simulink model "Code_Gen_Model"  (R2023b)
settings: Solver=FixedStepDiscrete  StartTime=0.0  StopTime=inf  FixedStep=t_sample  RelTol=1e-3
settings Model: Creator=FIRSTMentor
settings OptimizationCC: DefaultParameterBehavior=Inlined  StrengthReduction=on  PassReuseOutputArgsAs=Individual arguments  ZeroExternalMemoryAtStartup=off  ZeroInternalMemoryAtStartup=off  OptimizeBlockOrder=speed  OptimizationPriority=Speed  OptimizationCustomize=off  MultiThreadedLoops=on  EfficientTunableParamExpr=on
settings DebuggingCC: MergeDetectMultiDrivingBlocksExec=none  ParameterTunabilityLossMsg=error
settings ModelReferenceCC: PropagateSignalLabelsOutOfModel=off
settings SFSimCC: MATLABDynamicMemAlloc=off
settings RTWCC: Description=Embedded Coder  SystemTargetFile=ert.tlc  GenCodeOnly=on  TemplateMakefile=ert_default_tmf  Toolchain=MinGW64 | gmake (64-bit Windows)
settings CodeAppCC: ForceParamTrailComments=on  IgnoreCustomStorageClasses=off  OperatorAnnotations=on  SimulinkDataObjDesc=on  SFDataObjDesc=on  InsertBlockDesc=on
settings ERTTargetCC: TargetLangStandard=C99 (ISO)  GenerateSampleERTMain=on  ParenthesesLevel=Minimum  InlinedParameterPlacement=NonHierarchical  ERTCustomFileTemplate=example_file_process.tlc

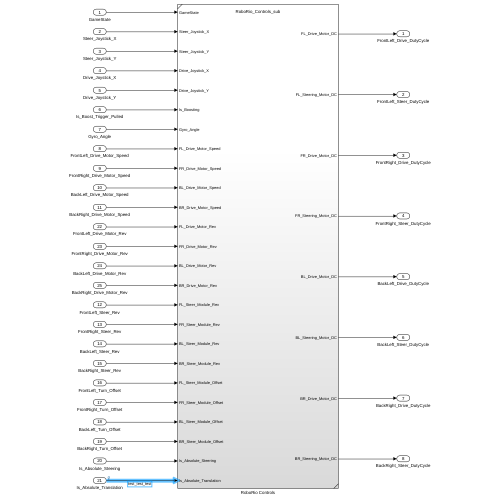
[thumbnail: Simulink's stored preview of the top-level diagram]
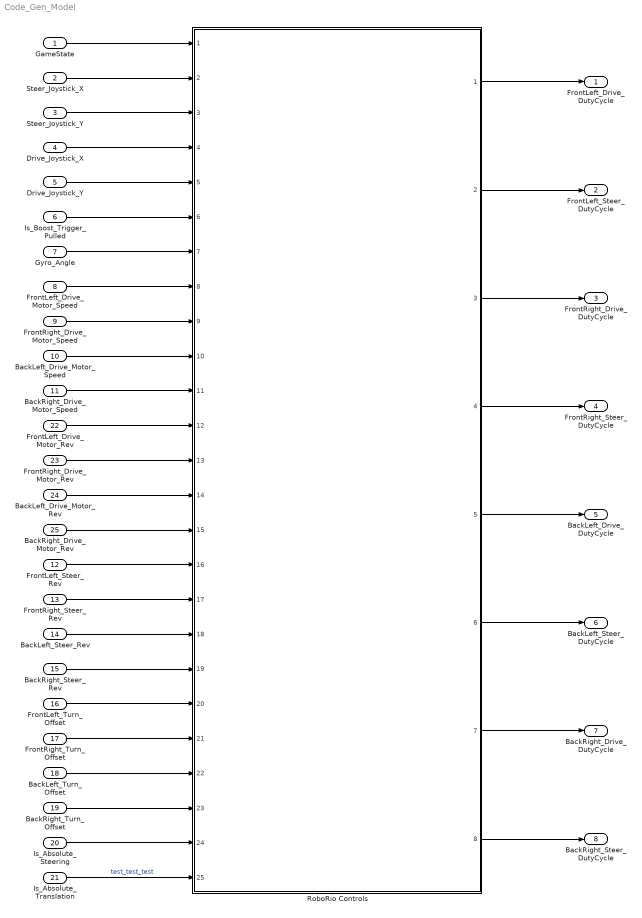
== system Code_Gen_Model ==
  GameState : Inport
  Steer_Joystick_X : Inport  Port=2
  Steer_Joystick_Y : Inport  Port=3
  Drive_Joystick_X : Inport  Port=4
  Drive_Joystick_Y : Inport  Port=5
  Is_Boost_Trigger_Pulled : Inport  Port=6
  Gyro_Angle : Inport  Port=7
  FrontLeft_Drive_Motor_Speed : Inport  Port=8
  FrontRight_Drive_Motor_Speed : Inport  Port=9
  BackLeft_Drive_Motor_Speed : Inport  Port=10
  BackRight_Drive_Motor_Speed : Inport  Port=11
  FrontLeft_Steer_Rev : Inport  Port=12
  FrontRight_Steer_Rev : Inport  Port=13
  BackLeft_Steer_Rev : Inport  Port=14
  BackRight_Steer_Rev : Inport  Port=15
  FrontLeft_Turn_Offset : Inport  Port=16
  FrontRight_Turn_Offset : Inport  Port=17
  BackLeft_Turn_Offset : Inport  Port=18
  BackRight_Turn_Offset : Inport  Port=19
  Is_Absolute_Steering : Inport  Port=20
  Is_Absolute_Translation : Inport  Port=21
  FrontLeft_Drive_Motor_Rev : Inport  Port=22
  FrontRight_Drive_Motor_Rev : Inport  Port=23
  BackLeft_Drive_Motor_Rev : Inport  Port=24
  BackRight_Drive_Motor_Rev : Inport  Port=25
  RoboRio Controls : Subsystem  ReferencedSubsystem=RoboRio_Controls_sub
  FrontLeft_Drive_DutyCycle : Outport
  FrontLeft_Steer_DutyCycle : Outport  Port=2
  FrontRight_Drive_DutyCycle : Outport  Port=3
  FrontRight_Steer_DutyCycle : Outport  Port=4
  BackLeft_Drive_DutyCycle : Outport  Port=5
  BackLeft_Steer_DutyCycle : Outport  Port=6
  BackRight_Drive_DutyCycle : Outport  Port=7
  BackRight_Steer_DutyCycle : Outport  Port=8
  wires:
  RoboRio Controls/7 -> BackRight_Drive_DutyCycle/1
  Drive_Joystick_X/1 -> RoboRio Controls/4
  Is_Absolute_Steering/1 -> RoboRio Controls/24
  Steer_Joystick_X/1 -> RoboRio Controls/2
  RoboRio Controls/3 -> FrontRight_Drive_DutyCycle/1
  BackRight_Turn_Offset/1 -> RoboRio Controls/23
  GameState/1 -> RoboRio Controls/1
  RoboRio Controls/4 -> FrontRight_Steer_DutyCycle/1
  Is_Boost_Trigger_Pulled/1 -> RoboRio Controls/6
  FrontLeft_Drive_Motor_Speed/1 -> RoboRio Controls/8
  RoboRio Controls/6 -> BackLeft_Steer_DutyCycle/1
  BackLeft_Steer_Rev/1 -> RoboRio Controls/18
  Gyro_Angle/1 -> RoboRio Controls/7
  FrontRight_Steer_Rev/1 -> RoboRio Controls/17
  Steer_Joystick_Y/1 -> RoboRio Controls/3
  Drive_Joystick_Y/1 -> RoboRio Controls/5
  RoboRio Controls/2 -> FrontLeft_Steer_DutyCycle/1
  FrontRight_Drive_Motor_Speed/1 -> RoboRio Controls/9
  BackLeft_Drive_Motor_Speed/1 -> RoboRio Controls/10
  BackLeft_Turn_Offset/1 -> RoboRio Controls/22
  BackRight_Drive_Motor_Speed/1 -> RoboRio Controls/11
  FrontLeft_Drive_Motor_Rev/1 -> RoboRio Controls/12
  Is_Absolute_Translation/1 -> RoboRio Controls/25  "test_test_test"
  BackRight_Steer_Rev/1 -> RoboRio Controls/19
  FrontRight_Drive_Motor_Rev/1 -> RoboRio Controls/13
  BackLeft_Drive_Motor_Rev/1 -> RoboRio Controls/14
  BackRight_Drive_Motor_Rev/1 -> RoboRio Controls/15
  FrontLeft_Steer_Rev/1 -> RoboRio Controls/16
  RoboRio Controls/8 -> BackRight_Steer_DutyCycle/1
  FrontLeft_Turn_Offset/1 -> RoboRio Controls/20
  FrontRight_Turn_Offset/1 -> RoboRio Controls/21
  RoboRio Controls/1 -> FrontLeft_Drive_DutyCycle/1
  RoboRio Controls/5 -> BackLeft_Drive_DutyCycle/1
